simulink model "smMarsRover"  (R2024b)
settings: Solver=VariableStepAuto  StartTime=0.0  StopTime=51  RelTol=1e-3
PreLoadFcn:
  | run_sm
values from neighbouring files (symbols this model uses):
  arm_q0 = [-2.3554 -125.9144   49.8193 -175.7336  177.6446  180.0000]    [sm_mars_rover_params.m]
  goal_loc = [roverPath.x(end) roverPath.y(end)]    [sm_mars_rover_params.m]
  Z = fillmissing(Z, 'linear')    [setup.m]
undefined symbols (not defined in the file or in its folder): cameraData, Chassis_L, Chassis_width, eeConfig, Kd, Kd_arm, Kd_steer, Ki, Ki_arm, Ki_steer, Kp, Kp_arm, Kp_steer, Link1, Link2, Link3, R_disc_Link1, rover_accel, roverPath, t1, TrqLoLimit, TrqUpLimit, Wheel1_G, Wheel2_G, Wheel3_G, Wheel4_G, Wheel5_G, Wheel6_G, Wheel_Radius, X, Y
libraries: sm_lib x216, nesl_utility x51, slpidlib x3, simulink x3, robotcorelib x1, robotalgslib x1, simulink_extras x1
(part 1 of 7)
settings Model: Creator=dipayan  LastModifiedBy=dipayan

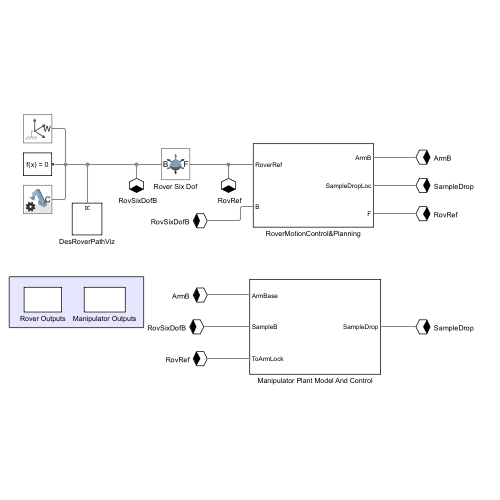
[thumbnail: Simulink's stored preview of the top-level diagram]
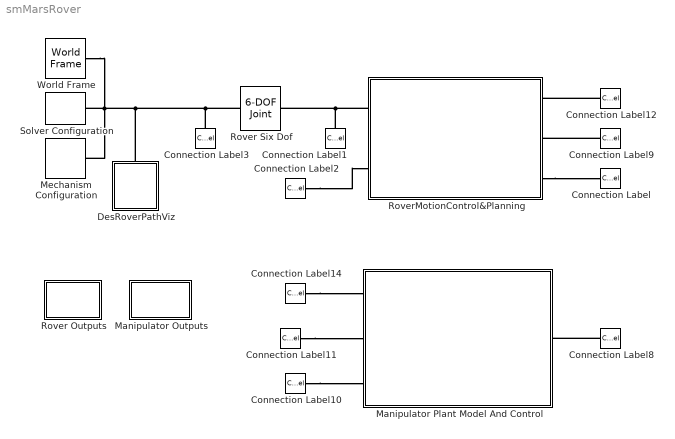
== system smMarsRover ==
  Connection Label : ConnectionLabel  Label=RovRef
  Connection Label1 : ConnectionLabel  Label=RovRef
  Connection Label10 : ConnectionLabel  Label=RovRef
  Connection Label11 : ConnectionLabel  Label=RovSixDofB
  Connection Label12 : ConnectionLabel  Label=ArmB
  Connection Label14 : ConnectionLabel  Label=ArmB
  Connection Label2 : ConnectionLabel  Label=RovSixDofB
  Connection Label3 : ConnectionLabel  Label=RovSixDofB
  Connection Label8 : ConnectionLabel  Label=SampleDrop
  Connection Label9 : ConnectionLabel  Label=SampleDrop
  DesRoverPathViz : Subsystem
  Manipulator Outputs : Subsystem
  Manipulator Plant Model And Control : Subsystem
  Mechanism Configuration : sm_lib/Utilities/Mechanism Configuration  UniformGravity=Constant  GravityVector=[0 0 -3.72076]  GravityVectorUnits=m/s^2  LinearizationDelta=0.001  JointModeTransitionNonlinearIterations=2
  Rover Outputs : Subsystem
  Rover Six Dof : sm_lib/Joints/6-DOF Joint  JointMode=Normal  CompositeWrenchDir=FollowerOnBase  CompositeWrenchFrame=BaseFrame  SenseConstraintForce=off  SenseConstraintTorque=off  SenseTotalForce=off  SenseTotalTorque=off  PxPositionTargetSpecify=on  PxPositionTargetPriority=High  PxPositionTargetValue=roverPath.x(1)  PxPositionTargetValueUnits=m  PxVelocityTargetSpecify=off  PxVelocityTargetPriority=High  PxVelocityTargetValue=0  PxVelocityTargetValueUnits=m/s  PxEquilibriumPosition=0  PxEquilibriumPositionUnits=m  PxSpringStiffness=0  PxSpringStiffnessUnits=N/m  PxDampingCoefficient=0  PxDampingCoefficientUnits=N/(m/s)  PxLowerLimitSpecify=off  PxLowerLimitBound=-1  PxLowerLimitBoundUnits=m  PxLowerLimitStiffness=1e6  PxLowerLimitStiffnessUnits=N/m  PxLowerLimitDamping=1e3  PxLowerLimitDampingUnits=N/(m/s)  PxLowerLimitTransitionRegionWidth=1e-4  PxLowerLimitTransitionRegionWidthUnits=m  PxUpperLimitSpecify=off  PxUpperLimitBound=1  PxUpperLimitBoundUnits=m  PxUpperLimitStiffness=1e6  PxUpperLimitStiffnessUnits=N/m  PxUpperLimitDamping=1e3  PxUpperLimitDampingUnits=N/(m/s)  PxUpperLimitTransitionRegionWidth=1e-4  PxUpperLimitTransitionRegionWidthUnits=m  PxTorqueActuationMode=NoTorque  PxMotionActuationMode=ComputedMotion  PxSensePosition=off  PxSenseVelocity=off  PxSenseAcceleration=off  PxSenseTorqueForce=off  PxSenseLowerLimitTorqueForce=off  PxSenseUpperLimitTorqueForce=off  PyPositionTargetSpecify=on  PyPositionTargetPriority=High  PyPositionTargetValue=roverPath.y(1)  PyPositionTargetValueUnits=m  PyVelocityTargetSpecify=off  PyVelocityTargetPriority=High  PyVelocityTargetValue=-2  PyVelocityTargetValueUnits=m/s  PyEquilibriumPosition=0  PyEquilibriumPositionUnits=m  PySpringStiffness=0  PySpringStiffnessUnits=N/m  PyDampingCoefficient=0  PyDampingCoefficientUnits=N/(m/s)  PyLowerLimitSpecify=off  PyLowerLimitBound=-1  PyLowerLimitBoundUnits=m  PyLowerLimitStiffness=1e6  PyLowerLimitStiffnessUnits=N/m  PyLowerLimitDamping=1e3  PyLowerLimitDampingUnits=N/(m/s)  PyLowerLimitTransitionRegionWidth=1e-4  PyLowerLimitTransitionRegionWidthUnits=m  PyUpperLimitSpecify=off  PyUpperLimitBound=1  PyUpperLimitBoundUnits=m  PyUpperLimitStiffness=1e6  PyUpperLimitStiffnessUnits=N/m  PyUpperLimitDamping=1e3  PyUpperLimitDampingUnits=N/(m/s)  PyUpperLimitTransitionRegionWidth=1e-4  PyUpperLimitTransitionRegionWidthUnits=m  PyTorqueActuationMode=NoTorque  PyMotionActuationMode=ComputedMotion  PySensePosition=off  PySenseVelocity=off  PySenseAcceleration=off  PySenseTorqueForce=off  PySenseLowerLimitTorqueForce=off  PySenseUpperLimitTorqueForce=off  PzPositionTargetSpecify=on  PzPositionTargetPriority=High  PzPositionTargetValue=roverPath.t0.pzOffset  PzPositionTargetValueUnits=m  PzVelocityTargetSpecify=off  PzVelocityTargetPriority=High  PzVelocityTargetValue=0  PzVelocityTargetValueUnits=m/s  PzEquilibriumPosition=0  PzEquilibriumPositionUnits=m  PzSpringStiffness=0  PzSpringStiffnessUnits=N/m  PzDampingCoefficient=0  PzDampingCoefficientUnits=N/(m/s)  PzLowerLimitSpecify=off  PzLowerLimitBound=-1  PzLowerLimitBoundUnits=m  PzLowerLimitStiffness=1e6  PzLowerLimitStiffnessUnits=N/m  PzLowerLimitDamping=1e3  PzLowerLimitDampingUnits=N/(m/s)  PzLowerLimitTransitionRegionWidth=1e-4  PzLowerLimitTransitionRegionWidthUnits=m  PzUpperLimitSpecify=off  PzUpperLimitBound=1  PzUpperLimitBoundUnits=m  PzUpperLimitStiffness=1e6  PzUpperLimitStiffnessUnits=N/m  PzUpperLimitDamping=1e3  PzUpperLimitDampingUnits=N/(m/s)  PzUpperLimitTransitionRegionWidth=1e-4  PzUpperLimitTransitionRegionWidthUnits=m  PzTorqueActuationMode=NoTorque  PzMotionActuationMode=ComputedMotion  PzSensePosition=off  PzSenseVelocity=off  PzSenseAcceleration=off  PzSenseTorqueForce=off  PzSenseLowerLimitTorqueForce=off  PzSenseUpperLimitTorqueForce=off  SphPositionTargetSpecify=on  SphPositionTargetPriority=High  SphPositionTargetRotationMethod=RotationSequence  SphPositionTargetFollAlignAxisA=+X  SphPositionTargetBaseAlignAxisA=+Y  SphPositionTargetFollAlignAxisB=+Y  SphPositionTargetBaseAlignAxisB=+Z  SphPositionTargetRotationStandardAxis=+X  SphPositionTargetRotationAngle=5  SphPositionTargetRotationAngleUnits=deg  SphPositionTargetRotationArbitraryAxis=[0 0 1]  SphPositionTargetRotationSequenceAxes=FollowerAxes  SphPositionTargetRotationSequence=ZYX  SphPositionTargetRotationSequenceAngles=[roverPath.t0.yaw, roverPath.t0.pitch, roverPath.t0.roll]  SphPositionTargetRotationSequenceAnglesUnits=rad  SphPositionTargetRotationMatrix=[1 0 0; 0 1 0; 0 0 1]  SphPositionTargetQuaternion=[1 0 0 0]  SphVelocityTargetSpecify=off  SphVelocityTargetPriority=High  SphVelocityTargetValue=[0 0 45]  SphVelocityTargetValueUnits=deg/s  SphVelocityTargetInFollowerFrame=on  SphEqPosRotationMethod=None  SphEqPosFollAlignAxisA=+X  SphEqPosBaseAlignAxisA=+Y  SphEqPosFollAlignAxisB=+Y  SphEqPosBaseAlignAxisB=+Z  SphEqPosRotationStandardAxis=+Z  SphEqPosRotationAngle=0.0  SphEqPosRotationAngleUnits=deg  SphEqPosRotationArbitraryAxis=[0 0 1]  SphEqPosRotationSequenceAxes=FollowerAxes  SphEqPosRotationSequence=XYX  SphEqPosRotationSequenceAngles=[0 0 0]  SphEqPosRotationSequenceAnglesUnits=deg  SphEqPosRotationMatrix=[1 0 0; 0 1 0; 0 0 1]  SphEqPosQuaternion=[1 0 0 0]  SphSpringStiffness=0  SphSpringStiffnessUnits=m*N/deg  SphDampingCoefficient=0  SphDampingCoefficientUnits=m*s*N/deg  SphLowerLimitSpecify=off  SphLowerLimitBound=15  SphLowerLimitBoundUnits=deg  SphLowerLimitStiffness=1e4  SphLowerLimitStiffnessUnits=N*m/deg  SphLowerLimitDamping=10  SphLowerLimitDampingUnits=N*m/(deg/s)  SphLowerLimitTransitionRegionWidth=0.1  SphLowerLimitTransitionRegionWidthUnits=deg  SphUpperLimitSpecify=off  SphUpperLimitBound=45  SphUpperLimitBoundUnits=deg  SphUpperLimitStiffness=1e4  SphUpperLimitStiffnessUnits=N*m/deg  SphUpperLimitDamping=10  SphUpperLimitDampingUnits=N*m/(deg/s)  SphUpperLimitTransitionRegionWidth=0.1  SphUpperLimitTransitionRegionWidthUnits=deg  SphTorqueActuationMode=NoTorque  SphActuateTorqueX=off  SphActuateTorqueY=off  SphActuateTorqueZ=off  SphActuateTorque=off  SphActuationFrame=BaseFrame  SphSensePosition=off  SphSenseVelocityX=off  SphSenseVelocityY=off  SphSenseVelocityZ=off  SphSenseVelocity=off  SphSenseAccelerationX=off  SphSenseAccelerationY=off  SphSenseAccelerationZ=off  SphSenseAcceleration=off  SphSenseLowerLimitTorqueMag=off  SphSenseUpperLimitTorqueMag=off  SphSensingFrame=FollowerFrame
  RoverMotionControl&Planning : Subsystem
  Solver Configuration : nesl_utility/Solver Configuration  PhysicalDomain=network_engine_domain  SubClassName=solver  LeftPortType=input  RightPortType=generic  Tones=[]  Harmonics=[]  SimulateNoise=off  Profile=off  UseLocalSampling=off  EnableSwitchedLinearOptims=on  FrequencyDomain=off  UseCCode=off  RelTol=0.001  AbsTol=1e-06  MinStep=1e-09  ToWorkspace=off  RevertToSquareIcSolve=off  NumHomotopyIterations=100  PhasorMode=off  PhasorModeNumHarmonics=1  ConsistencySolver=NEWTON_FTOL  IndexReductionMethod=DerivativeReplacement  DoDC=off  ResidualTolerance=1e-09  ConsistencyTolSource=GLOBAL  ConsistencyAbsTol=0.001  ConsistencyRelTol=0.001  ConsistencyTolFactor=0.001  UseLocalSolver=off  LocalSolverChoice=NE_BACKWARD_EULER_ADVANCER  ResolveIndetEquations=on  FunctionEvalNumThread=1  LocalSolverSampleTime=0.001  DoFixedCost=off  MaxNonlinIter=3  MaxModeIter=2  ComputeImpulses=off  ImpulseIterations=2  LinearAlgebra=auto  LinearAlgebraNumThread=0  EquationFormulation=NE_TIME_EF  DelaysMemoryBudget=1024  AutomaticFiltering=on  FilteringTimeConstant=0.001  PartitionStorageMethod=AS_NEEDED  PartitionMemoryBudget=1024  PartitionMethod=FAST  MultibodyUseLocalSolver=off  MultibodyLocalSolverChoice=ODE1  MultibodyLocalSolverSampleTime=0.001
  World Frame : sm_lib/Frames and Transforms/World Frame
  connections:
  Solver Configuration/RConn1 -- Connection Label3/LConn1 -- Rover Six Dof/LConn1 -- DesRoverPathViz/LConn1 -- World Frame/RConn1 -- Mechanism Configuration/RConn1
  RoverMotionControl&Planning/LConn1 -- Connection Label1/LConn1 -- Rover Six Dof/RConn1
  RoverMotionControl&Planning/RConn3 -- Connection Label/LConn1
  Connection Label12/LConn1 -- RoverMotionControl&Planning/RConn1
  Connection Label9/LConn1 -- RoverMotionControl&Planning/RConn2
  Connection Label2/LConn1 -- RoverMotionControl&Planning/LConn2
  Connection Label14/LConn1 -- Manipulator Plant Model And Control/LConn1
  Connection Label11/LConn1 -- Manipulator Plant Model And Control/LConn2
  Connection Label10/LConn1 -- Manipulator Plant Model And Control/LConn3
  Connection Label8/LConn1 -- Manipulator Plant Model And Control/RConn1

== system smMarsRover/DesRoverPathViz ==
  Desired Path Viz : sm_lib/Curves and Surfaces/Point Cloud  CoordinatesMatrix=pointCloud  CoordinatesMatrixUnits=m  GraphicType=MarkerCloud  GraphicSphereRadius=0.05  GraphicSphereRadiusUnits=m  GraphicVisPropType=SimpleVisualProperties  GraphicDiffuseColor=[0 0 1]  GraphicOpacity=0.5  GraphicSpecularColor=[0.5 0.5 0.5 1.0]  GraphicAmbientColor=[0.15 0.15 0.15 1.0]  GraphicEmissiveColor=[0.0 0.0 0.0 1.0]  GraphicShininess=75
  Rigid Transform6 : sm_lib/Frames and Transforms/Rigid Transform  RotationMethod=None  FollAlignAxisA=+X  BaseAlignAxisA=+Y  FollAlignAxisB=+Y  BaseAlignAxisB=+Z  RotationStandardAxis=+X  RotationAngle=90  RotationAngleUnits=deg  RotationArbitraryAxis=[0 0 1]  RotationSequenceAxes=FollowerAxes  RotationSequence=XYX  RotationSequenceAngles=[0 0 0]  RotationSequenceAnglesUnits=deg  RotationMatrix=[1 0 0; 0 1 0; 0 0 1]  Quaternion=[1 0 0 0]  TranslationMethod=Cartesian  TranslationCartesianOffset=[0 0 roverPath.Offset_vis_z]  TranslationCartesianOffsetUnits=m  TranslationStandardAxis=+Z  TranslationStandardOffset=1.85  TranslationStandardOffsetUnits=m  TranslationROffset=0  TranslationROffsetUnits=m  TranslationThetaOffset=0  TranslationThetaOffsetUnits=deg  TranslationZOffset=0  TranslationZOffsetUnits=m
  Spline : sm_lib/Curves and Surfaces/Spline  DataPoints=pointCloud  DataPointsUnits=m  EndConditionType=Natural  GraphicType=FromGeometry  MarkerShape=Sphere  MarkerSize=10  GraphicVisPropType=SimpleVisualProperties  GraphicDiffuseColor=[0 0.4471 0.7412]  GraphicOpacity=0.5  GraphicSpecularColor=[0.5 0.5 0.5 1.0]  GraphicAmbientColor=[0.15 0.15 0.15 1.0]  GraphicEmissiveColor=[0.0 0.0 0.0 1.0]  GraphicShininess=75
  R : PMIOPort  Side=Left
  connections:
  Desired Path Viz/LConn1 -- Rigid Transform6/RConn1 -- Spline/LConn1
  R/RConn1 -- Rigid Transform6/LConn1

== system smMarsRover/Manipulator Outputs ==
  ManipulatorJointActuatorTrqs : Scope  NumInputPorts=6
  ManipulatorJointAngles : Scope  NumInputPorts=6
  SelectSignal4 : Subsystem
  SelectSignal5 : Subsystem
  wires:
  SelectSignal4/5(Out4) -> ManipulatorJointAngles/5
  SelectSignal5/3(Out3) -> ManipulatorJointActuatorTrqs/3
  SelectSignal4/2(Out2) -> ManipulatorJointAngles/2
  SelectSignal4/1(Out1) -> ManipulatorJointAngles/1
  SelectSignal5/2(Out2) -> ManipulatorJointActuatorTrqs/2
  SelectSignal4/6(Out6) -> ManipulatorJointAngles/6
  SelectSignal5/4(Out5) -> ManipulatorJointActuatorTrqs/4
  SelectSignal4/3(Out3) -> ManipulatorJointAngles/3
  SelectSignal5/1(Out1) -> ManipulatorJointActuatorTrqs/1
  SelectSignal5/5(Out4) -> ManipulatorJointActuatorTrqs/5
  SelectSignal4/4(Out5) -> ManipulatorJointAngles/4
  [DesiredJointAngles] -> SelectSignal4/1(In1)
  [JointActuatorTrqs] -> SelectSignal5/1(In1)
  [ActJointAngles] -> SelectSignal4/2(In2)
  SelectSignal5/6(Out6) -> ManipulatorJointActuatorTrqs/6

== system smMarsRover/Manipulator Plant Model And Control ==
  " Trajectory Planner" : Subsystem
  Add : Sum  Inputs=+-
  ArmLock : Subsystem
  End Effector Sense : Subsystem
  PID Control : slpidlib/PID Controller  Controller=PID  Form=Parallel  TimeDomain=Continuous-time  UseExternalTs=off  SampleTime=-1  IntegratorMethod=Forward Euler  FilterMethod=Forward Euler  ControllerParametersSource=internal  P=Kp_arm  I=Ki_arm  UseKiTs=off  D=Kd_arm  UseExternalDerivativeSource=off  N=100  UseFilter=on  TunerSelectOption=Transfer Function Based (PID Tuner App)  InitialConditionSource=internal  InitialConditionForIntegrator=0  InitialConditionForFilter=0  DifferentiatorICPrevScaledInput=0  ExternalReset=none  TrackingMode=off  Kt=1  LimitOutput=off  SatLimitsSource=internal  UpperSaturationLimit=inf  LowerSaturationLimit=-inf  LinearizeAsGain=on  AntiWindupMode=none  Kb=1  LimitIntegrator=off  UpperIntegratorSaturationLimit=inf  LowerIntegratorSaturationLimit=-inf  POutMin=[]  POutMax=[]  IOutMin=[]  IOutMax=[]  DOutMin=[]  DOutMax=[]  NOutMin=[]  NOutMax=[]  SumOutMin=[]  SumOutMax=[]  SaturationOutMin=[]  SaturationOutMax=[]  PParamMin=[]  PParamMax=[]  IParamMin=[]  IParamMax=[]  DParamMin=[]  DParamMax=[]  NParamMin=[]  NParamMax=[]  KbParamMin=[]  KbParamMax=[]  KtParamMin=[]  KtParamMax=[]  KbOutMin=[]  KbOutMax=[]  KtOutMin=[]  KtOutMax=[]  IntegratorOutMin=[]  IntegratorOutMax=[]  FilterOutMin=[]  FilterOutMax=[]  SumI1OutMin=[]  SumI1OutMax=[]  SumI2OutMin=[]  SumI2OutMax=[]  SumI3OutMin=[]  SumI3OutMax=[]  SumI4OutMin=[]  SumI4OutMax=[]  SumDOutMin=[]  SumDOutMax=[]  DifferentiatorOutMin=[]  DifferentiatorOutMax=[]  FilterDiffOutCoefMin=[]  FilterDiffOutCoefMax=[]  ReciprocalOutMin=[]  ReciprocalOutMax=[]  SumDenOutMin=[]  SumDenOutMax=[]  SumNumOutMin=[]  SumNumOutMax=[]  DivideOutMin=[]  DivideOutMax=[]  UdiffTsProdOutMin=[]  UdiffTsProdOutMax=[]  NTsProdOutMin=[]  NTsProdOutMax=[]  UintegralTsProdOutMin=[]  UintegralTsProdOutMax=[]  UngainTsProdOutMin=[]  UngainTsProdOutMax=[]  ClampingZeroOutDataTypeStr=Inherit: Inherit via back propagation  ClampingZeroOutMin=[]  ClampingZeroOutMax=[]  FilterDenConstantOutDataTypeStr=Inherit: Inherit via back propagation  FilterDenConstantOutMin=[]  FilterDenConstantOutMax=[]  PCopyOutDataTypeStr=Inherit: Inherit via back propagation  PCopyOutMin=[]  PCopyOutMax=[]  NCopyOutDataTypeStr=Inherit: Inherit via back propagation  NCopyOutMin=[]  NCopyOutMax=[]  IntegratorContinuousStateAttributes=''  IntegratorStateMustResolveToSignalObject=off  IntegratorRTWStateStorageClass=Auto  FilterContinuousStateAttributes=''  FilterStateMustResolveToSignalObject=off  FilterRTWStateStorageClass=Auto  ParallelPVariant=InternalParameters  IdealPVariant=Disabled  IVariant=InternalParameters  DVariant=InternalParameters  IntegratorVariant=Continuous  SatVariant=Disabled  AWVariant=Passthrough  PCopyVariant=Disabled  TRVariant=Disabled  FdbkBlocksVariant=Forward  IdealPFdbkVariant=Disabled  SatFdbkVariant=Disabled  DerivativeFilterVariant=ContFilter  NVariant=InternalParameters  NCopyVariant=Disabled  FilterICVariant=InternalICsFilter  IntegratorICVariant=InternalICs  ExternalResetVariant=Disabled  TRSumVariant=Passthrough  SumFdbkVariant=Disabled  SumVariant=Sum_PID  TsampFilterVariant=InternalTs  TsampNgainVariant=Passthrough  TsampIntegralVariant=Disabled_SignalSpec  ExternalSaturationOutDataTypeStr=Inherit: Same as second input  DerivativeSourceVariant=ErrorSignal  PreIntVariant=InternalPreInt
  Rover Arm : Subsystem
      settings: PortSchema="{\"entries\":[{\"content\":{\"sides\":[{\"content\":{\"connectorIds\":[\"In1\"]},\"type\":\"ConnectorPlacement.EquallySpacedRectSide\",\"uuid\":\"44c8adb7-00ac-400a-98ed-ead5e12ad105\"},{\"content\":{\"connectorIds\":[\"Out1\"],\"side\":\"RIGHT\"},\"type\":\"ConnectorPlacement.EquallySpacedRectSide\",\"uuid\":\"fdc7bd8f-ace2-488d-8919-cf5c650dd1d7\"},{\"content\":{\"connectorIds\":[\"LConn1\",\"LConn2\"],\"side\":\"TOP\"},\"type\":\"ConnectorPlacement.EquallySpacedRectSide\",\"uuid\":\"e6b89b0c-12bb-4698-b60e-60c64a8f3314\"}]},\"type\":\"ConnectorPlacement.EquallySpacedConnector\",\"uuid\":\"42e45278-5e8a-4850-9160-494ec176052c\"}],\"packageUris\":[\"http://schema.mathworks.com/mf0/Connector/R2020b\"],\"version\":\"1.0\"}"
      mask Display: image('rover_manip_subsys_1.JPG');
  Sample Interaction Logic : Subsystem
      mask Display: image('sample_1.JPG');
  Sample Loc Sense : Subsystem
  ArmBase : PMIOPort  Side=Left
  SampleB : PMIOPort  Port=2  Side=Left
  ToArmLock : PMIOPort  Port=3  Side=Left
  SampleDrop : PMIOPort  Port=4  Side=Right
  tag scope: ActJointAngles=global, DesiredJointAngles=global, JointActuatorTrqs=global
  wires:
  Add/1 -> PID Control/1
  Rover Arm/1(JointAngles) -> " Trajectory Planner"/2(ActJointAngles), Add/2, [ActJointAngles]
  " Trajectory Planner"/1(DesiredJointAngles) -> [DesiredJointAngles], Add/1
  PID Control/1 -> [JointActuatorTrqs], Rover Arm/1(ActuatorTrqs)
  Sample Loc Sense/1(SamplePos) -> " Trajectory Planner"/1(SampleLocation)
  connections:
  Rover Arm/LConn2 -- Sample Interaction Logic/LConn2 -- ArmLock/RConn1 -- End Effector Sense/RConn1
  Rover Arm/LConn1 -- ArmBase/RConn1 -- Sample Loc Sense/LConn1 -- End Effector Sense/LConn1
  SampleB/RConn1 -- Sample Interaction Logic/LConn3
  Sample Loc Sense/RConn1 -- Sample Interaction Logic/LConn1
  SampleDrop/RConn1 -- Sample Interaction Logic/RConn1
  ToArmLock/RConn1 -- ArmLock/LConn1

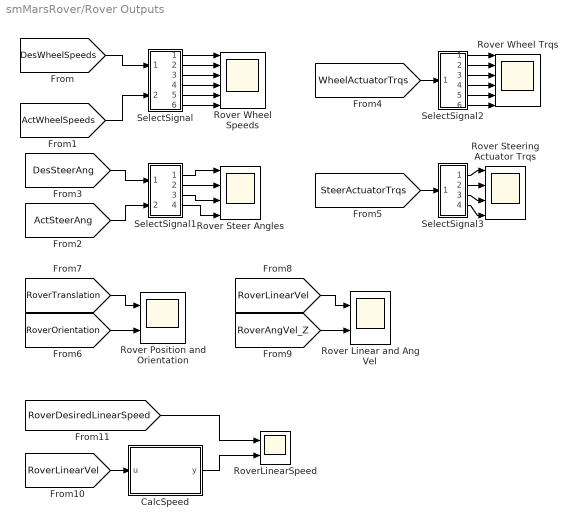
== system smMarsRover/Rover Outputs ==
  CalcSpeed : MATLAB Function  TreatAsAtomicUnit=on
  Rover Linear and Ang Vel : Scope  NumInputPorts=2
  Rover Position and Orientation : Scope  NumInputPorts=2
  Rover Steer Angles : Scope  NumInputPorts=4
  Rover Steering Actuator Trqs : Scope  NumInputPorts=4
  Rover Wheel Speeds : Scope  NumInputPorts=6
  Rover Wheel Trqs : Scope  NumInputPorts=6
  RoverLinearSpeed : Scope  NumInputPorts=2
  SelectSignal : Subsystem
  SelectSignal1 : Subsystem
  SelectSignal2 : Subsystem
  SelectSignal3 : Subsystem
  wires:
  CalcSpeed/1(y) -> RoverLinearSpeed/2
  SelectSignal3/1(Out1) -> Rover Steering Actuator Trqs/1
  [RoverLinearVel] -> CalcSpeed/1(u)
  [RoverAngVel_Z] -> Rover Linear and Ang Vel/2
  [RoverLinearVel] -> Rover Linear and Ang Vel/1
  [DesWheelSpeeds] -> SelectSignal/1(In1)
  SelectSignal2/4(Out4) -> Rover Wheel Trqs/4
  [WheelActuatorTrqs] -> SelectSignal2/1(In1)
  SelectSignal1/2(Out2) -> Rover Steer Angles/2
  [RoverTranslation] -> Rover Position and Orientation/1
  SelectSignal3/2(Out2) -> Rover Steering Actuator Trqs/2
  SelectSignal3/3(Out3) -> Rover Steering Actuator Trqs/3
  [DesSteerAng] -> SelectSignal1/1(In1)
  SelectSignal2/3(Out3) -> Rover Wheel Trqs/3
  [RoverOrientation] -> Rover Position and Orientation/2
  SelectSignal3/4(Out5) -> Rover Steering Actuator Trqs/4
  SelectSignal2/6(Out6) -> Rover Wheel Trqs/6
  SelectSignal/3(Out3) -> Rover Wheel Speeds/3
  SelectSignal2/5(Out5) -> Rover Wheel Trqs/5
  SelectSignal/1(Out1) -> Rover Wheel Speeds/1
  SelectSignal/6(Out6) -> Rover Wheel Speeds/6
  [ActWheelSpeeds] -> SelectSignal/2(In2)
  SelectSignal2/1(Out1) -> Rover Wheel Trqs/1
  SelectSignal1/4(Out5) -> Rover Steer Angles/4
  [ActSteerAng] -> SelectSignal1/2(In2)
  SelectSignal/2(Out2) -> Rover Wheel Speeds/2
  [SteerActuatorTrqs] -> SelectSignal3/1(In1)
  SelectSignal/5(Out4) -> Rover Wheel Speeds/5
  SelectSignal2/2(Out2) -> Rover Wheel Trqs/2
  SelectSignal/4(Out5) -> Rover Wheel Speeds/4
  SelectSignal1/1(Out1) -> Rover Steer Angles/1
  SelectSignal1/3(Out3) -> Rover Steer Angles/3
  [RoverDesiredLinearSpeed] -> RoverLinearSpeed/1

== system smMarsRover/RoverMotionControl&Planning ==
  Rigid Terrain Surface : Subsystem
      mask Display: image('$imagefile'); % Use "Edit Image" on toolstrip to change.
  "Rover " : Subsystem
      settings: PortSchema="{\"entries\":[{\"content\":{\"sides\":[{\"content\":{\"connectorIds\":[\"LConn1\",\"In1\",\"In2\"]},\"type\":\"ConnectorPlacement.EquallySpacedRectSide\",\"uuid\":\"1e8a3e2b-b3ca-4467-863a-9c237d71771f\"},{\"content\":{\"connectorIds\":[\"RConn1\",\"RConn2\",\"RConn3\",\"Out1\",\"Out2\"],\"side\":\"RIGHT\"},\"type\":\"ConnectorPlacement.EquallySpacedRectSide\",\"uuid\":\"1c304fdb-ff64-4dc8-bd28-208b239a200a\"},{\"content\":{\"connectorIds\":[],\"side\":\"TOP\"},\"type\":\"ConnectorPlacement.EquallySpacedRectSide\",\"uuid\":\"6fd19973-5814-4525-bce6-20dd9c942e44\"}]},\"type\":\"ConnectorPlacement.EquallySpacedConnector\",\"uuid\":\"720db96a-3f3b-4ddd-a986-ea75ab459e47\"}],\"packageUris\":[\"http://schema.mathworks.com/mf0/Connector/R2020b\"],\"version\":\"1.0\"}"
      mask Display: image('$imagefile'); % Use "Edit Image" on toolstrip to change.
  Rover Path Planning And Control : Subsystem
  Rover Pose Sensing : Subsystem
  Steering Controller : Subsystem
  Wheel Speed Controller : Subsystem
  World Frame1 : sm_lib/Frames and Transforms/World Frame
  RoverRef : PMIOPort  Side=Left
  B : PMIOPort  Port=2  Side=Left
  ArmB : PMIOPort  Port=3  Side=Right
  SampleDropLoc : PMIOPort  Port=4  Side=Right
  F : PMIOPort  Port=5  Side=Right
  wires:
  "Rover "/1(ActSteerAng) -> Steering Controller/2(ActSteerAng)
  Rover Pose Sensing/1(Pose) -> Rover Path Planning And Control/1(CurrentPose)
  Rover Path Planning And Control/2(DesWheelSpeeds) -> Wheel Speed Controller/1(DesWheelSpeeds)
  "Rover "/2(ActWheelSpeeds) -> Wheel Speed Controller/2(ActWheelSpeed)
  Rover Pose Sensing/2(vSpeed) -> Rover Path Planning And Control/2(vSpeed)
  Steering Controller/1(SteerTrqs) -> "Rover "/1(SteeringTrqs)
  Rover Path Planning And Control/1(DesSteerAngs) -> Steering Controller/1(DesSteerAng)
  Wheel Speed Controller/1(WheelTrqs) -> "Rover "/2(WheelTrqs)
  connections:
  Rigid Terrain Surface/LConn1 -- "Rover "/RConn3
  SampleDropLoc/RConn1 -- "Rover "/RConn2
  B/RConn1 -- Rover Pose Sensing/LConn1
  World Frame1/RConn1 -- Rigid Terrain Surface/RConn1
  ArmB/RConn1 -- "Rover "/RConn1
  F/RConn1 -- Rover Pose Sensing/RConn1
  RoverRef/RConn1 -- "Rover "/LConn1

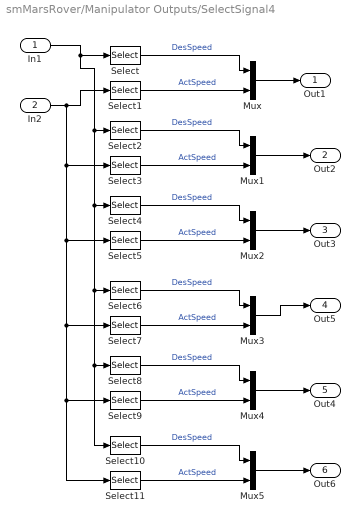
== system smMarsRover/Manipulator Outputs/SelectSignal4 ==
  In1 : Inport
  In2 : Inport  Port=2
  Mux{,1..5} (6 alike) : Mux  Inputs=2
  Select : Selector  InputPortWidth=6  IndexOptions=Index vector (dialog)  Indices=1  OutputSizes=1
  Select1 : Selector  InputPortWidth=6  IndexOptions=Index vector (dialog)  Indices=1  OutputSizes=1
  Select10 : Selector  InputPortWidth=6  IndexOptions=Index vector (dialog)  Indices=6  OutputSizes=1
  Select11 : Selector  InputPortWidth=6  IndexOptions=Index vector (dialog)  Indices=6  OutputSizes=1
  Select2 : Selector  InputPortWidth=6  IndexOptions=Index vector (dialog)  Indices=2  OutputSizes=1
  Select3 : Selector  InputPortWidth=6  IndexOptions=Index vector (dialog)  Indices=2  OutputSizes=1
  Select4 : Selector  InputPortWidth=6  IndexOptions=Index vector (dialog)  Indices=3  OutputSizes=1
  Select5 : Selector  InputPortWidth=6  IndexOptions=Index vector (dialog)  Indices=3  OutputSizes=1
  Select6 : Selector  InputPortWidth=6  IndexOptions=Index vector (dialog)  Indices=4  OutputSizes=1
  Select7 : Selector  InputPortWidth=6  IndexOptions=Index vector (dialog)  Indices=4  OutputSizes=1
  Select8 : Selector  InputPortWidth=6  IndexOptions=Index vector (dialog)  Indices=5  OutputSizes=1
  Select9 : Selector  InputPortWidth=6  IndexOptions=Index vector (dialog)  Indices=5  OutputSizes=1
  Out1 : Outport
  Out2 : Outport  Port=2
  Out3 : Outport  Port=3
  Out5 : Outport  Port=4
  Out4 : Outport  Port=5
  Out6 : Outport  Port=6
  wires:
  Select11/1 -> Mux5/2  "ActSpeed"
  Mux5/1 -> Out6/1
  Select10/1 -> Mux5/1  "DesSpeed"
  Select8/1 -> Mux4/1  "DesSpeed"
  Mux4/1 -> Out4/1
  Select9/1 -> Mux4/2  "ActSpeed"
  Select7/1 -> Mux3/2  "ActSpeed"
  Mux3/1 -> Out5/1
  Select6/1 -> Mux3/1  "DesSpeed"
  Select4/1 -> Mux2/1  "DesSpeed"
  Mux2/1 -> Out3/1
  Select5/1 -> Mux2/2  "ActSpeed"
  Select3/1 -> Mux1/2  "ActSpeed"
  Mux1/1 -> Out2/1
  Select2/1 -> Mux1/1  "DesSpeed"
  In2/1 -> Select1/1, Select3/1, Select5/1, Select7/1, Select9/1, Select11/1
  Select/1 -> Mux/1  "DesSpeed"
  In1/1 -> Select/1, Select2/1, Select4/1, Select6/1, Select8/1, Select10/1
  Mux/1 -> Out1/1
  Select1/1 -> Mux/2  "ActSpeed"

== system smMarsRover/Manipulator Outputs/SelectSignal5 ==
  In1 : Inport
  Select : Selector  InputPortWidth=6  IndexOptions=Index vector (dialog)  Indices=1  OutputSizes=1
  Select10 : Selector  InputPortWidth=6  IndexOptions=Index vector (dialog)  Indices=6  OutputSizes=1
  Select2 : Selector  InputPortWidth=6  IndexOptions=Index vector (dialog)  Indices=2  OutputSizes=1
  Select4 : Selector  InputPortWidth=6  IndexOptions=Index vector (dialog)  Indices=3  OutputSizes=1
  Select6 : Selector  InputPortWidth=6  IndexOptions=Index vector (dialog)  Indices=4  OutputSizes=1
  Select8 : Selector  InputPortWidth=6  IndexOptions=Index vector (dialog)  Indices=5  OutputSizes=1
  Transfer Fcn{1..6} (6 alike) : TransferFcn  Denominator=[0.1 1]
  Out1 : Outport
  Out2 : Outport  Port=2
  Out3 : Outport  Port=3
  Out5 : Outport  Port=4
  Out4 : Outport  Port=5
  Out6 : Outport  Port=6
  wires:
  Select10/1 -> Transfer Fcn5/1
  Select8/1 -> Transfer Fcn1/1
  Select6/1 -> Transfer Fcn2/1
  Select4/1 -> Transfer Fcn3/1
  Select2/1 -> Transfer Fcn4/1
  Select/1 -> Transfer Fcn6/1
  In1/1 -> Select10/1, Select8/1, Select6/1, Select4/1, Select2/1, Select/1
  Transfer Fcn6/1 -> Out1/1
  Transfer Fcn4/1 -> Out2/1
  Transfer Fcn3/1 -> Out3/1
  Transfer Fcn2/1 -> Out5/1
  Transfer Fcn1/1 -> Out4/1
  Transfer Fcn5/1 -> Out6/1

== system smMarsRover/Manipulator Plant Model And Control/ Trajectory Planner ==
  SampleLocation : Inport
  ActJointAngles : Inport  Port=2
  Constant : Constant  Value="[-2.2294 -125.2918   50.0575 -175.3493  177.7706  180.0000]"
  Delay : Delay
  Planner Subsystem : Subsystem
  SampleDropOffCmdLogic : Subsystem
  SampleLoc wrt arm base : Subsystem
  SamplePickUpCmdLogic : Subsystem
  Stop Simulation : Stop
  Switch : Switch  Criteria=u2 > Threshold  SaturateOnIntegerOverflow=off  InputSameDT=off
  DesiredJointAngles : Outport
  tag scope: ArmEnable=global, SampleDropOffFlag=global, SamplePickFlag=global
  wires:
  [RoverAtGoal] -> Planner Subsystem/Enable, Delay/1, SampleLoc wrt arm base/1(Enable)
  Switch/1 -> DesiredJointAngles/1
  Constant/1 -> Switch/3
  SampleDropOffCmdLogic/1(Out1) -> [SampleDropOffFlag]
  SamplePickUpCmdLogic/1(Out1) -> [SamplePickFlag]
  Delay/1 -> [ArmEnable], Switch/2
  ActJointAngles/1 -> Planner Subsystem/1(ActJointAngles)
  SampleLoc wrt arm base/1(SamplePos) -> Planner Subsystem/2(SamplePosition)
  Planner Subsystem/2(SamplePickCmd) -> SamplePickUpCmdLogic/1(u)
  Planner Subsystem/3(SampleDropCmd) -> SampleDropOffCmdLogic/1(u)
  [samplePickedSense] -> Planner Subsystem/3(IsSamplePicked)
  [sampleStoredSense] -> Planner Subsystem/4(IsSampleCollected)
  Planner Subsystem/1(DesJointAngles) -> Switch/1
  SampleLocation/1 -> SampleLoc wrt arm base/2(SampleLoc)
  Planner Subsystem/4(stop) -> Stop Simulation/1

== system smMarsRover/Manipulator Plant Model And Control/ArmLock ==
  note: Open arm lock by disengaging the Pristmatic joint when ArmEnable signal is true
  Constant1 : Constant  Value=-1
  Constant2 : Constant  Value=0
  Delay : Delay
  Rigid Transform : sm_lib/Frames and Transforms/Rigid Transform  RotationMethod=None  FollAlignAxisA=+X  BaseAlignAxisA=+Y  FollAlignAxisB=+Y  BaseAlignAxisB=+Z  RotationStandardAxis=+Z  RotationAngle=0.0  RotationAngleUnits=deg  RotationArbitraryAxis=[0 0 1]  RotationSequenceAxes=FollowerAxes  RotationSequence=XYX  RotationSequenceAngles=[0 0 0]  RotationSequenceAnglesUnits=deg  RotationMatrix=[1 0 0; 0 1 0; 0 0 1]  Quaternion=[1 0 0 0]  TranslationMethod=StandardAxis  TranslationCartesianOffset=[0 0 0]  TranslationCartesianOffsetUnits=m  TranslationStandardAxis=+Z  TranslationStandardOffset=-0.38  TranslationStandardOffsetUnits=m  TranslationROffset=0  TranslationROffsetUnits=m  TranslationThetaOffset=0  TranslationThetaOffsetUnits=deg  TranslationZOffset=0  TranslationZOffsetUnits=m
  Rigid Transform1 : sm_lib/Frames and Transforms/Rigid Transform  RotationMethod=StandardAxis  FollAlignAxisA=+X  BaseAlignAxisA=+Y  FollAlignAxisB=+Y  BaseAlignAxisB=+Z  RotationStandardAxis=+Z  RotationAngle=90  RotationAngleUnits=deg  RotationArbitraryAxis=[0 0 1]  RotationSequenceAxes=FollowerAxes  RotationSequence=XYX  RotationSequenceAngles=[0 0 0]  RotationSequenceAnglesUnits=deg  RotationMatrix=[1 0 0; 0 1 0; 0 0 1]  Quaternion=[1 0 0 0]  TranslationMethod=Cartesian  TranslationCartesianOffset=[0.6000 0.4853 0.3652]  TranslationCartesianOffsetUnits=m  TranslationStandardAxis=+Z  TranslationStandardOffset=0  TranslationStandardOffsetUnits=m  TranslationROffset=0  TranslationROffsetUnits=m  TranslationThetaOffset=0  TranslationThetaOffsetUnits=deg  TranslationZOffset=0  TranslationZOffsetUnits=m
  SPrismatic Joint : sm_lib/Joints/Prismatic Joint  JointMode=ProvidedByInput  CompositeWrenchDir=FollowerOnBase  CompositeWrenchFrame=BaseFrame  SenseConstraintForce=off  SenseConstraintTorque=off  SenseTotalForce=off  SenseTotalTorque=off  PositionTargetSpecify=off  PositionTargetPriority=High  PositionTargetValue=0  PositionTargetValueUnits=m  VelocityTargetSpecify=off  VelocityTargetPriority=High  VelocityTargetValue=0  VelocityTargetValueUnits=m/s  EquilibriumPosition=0  EquilibriumPositionUnits=m  SpringStiffness=0  SpringStiffnessUnits=N/m  DampingCoefficient=0  DampingCoefficientUnits=N/(m/s)  LowerLimitSpecify=on  LowerLimitBound=0  LowerLimitBoundUnits=m  LowerLimitStiffness=1e6  LowerLimitStiffnessUnits=N/m  LowerLimitDamping=1e3  LowerLimitDampingUnits=N/(m/s)  LowerLimitTransitionRegionWidth=1e-4  LowerLimitTransitionRegionWidthUnits=m  UpperLimitSpecify=off  UpperLimitBound=1  UpperLimitBoundUnits=m  UpperLimitStiffness=1e6  UpperLimitStiffnessUnits=N/m  UpperLimitDamping=1e3  UpperLimitDampingUnits=N/(m/s)  UpperLimitTransitionRegionWidth=1e-4  UpperLimitTransitionRegionWidthUnits=m  TorqueActuationMode=NoTorque  MotionActuationMode=ComputedMotion  SensePosition=off  SenseVelocity=off  SenseAcceleration=off  SenseTorqueForce=off  SenseLowerLimitTorqueForce=off  SenseUpperLimitTorqueForce=off
  Simulink-PS Converter : nesl_utility/Simulink-PS Converter  PhysicalDomain=network_engine_domain  SubClassName=ps_input  LeftPortType=input  RightPortType=output  PseudoPeriodic=off  Frequencies=[]  NoiseDistribution=none  NoiseParameters=[]  Unit=1  AffineConversion=off  FilteringAndDerivatives=provide  SimscapeFilterOrder=1  InputFilterTimeConstant=0.001  UdotUserProvided=0
  Switch1 : Switch  Criteria=u2 > Threshold  SaturateOnIntegerOverflow=off  InputSameDT=off
  Conn1 : PMIOPort  Side=Right
  Conn2 : PMIOPort  Port=2  Side=Left
  wires:
  Constant1/1 -> Switch1/1
  Switch1/1 -> Simulink-PS Converter/1
  Constant2/1 -> Switch1/3
  [ArmEnable] -> Delay/1
  Delay/1 -> Switch1/2
  connections:
  Rigid Transform1/LConn1 -- Rigid Transform/RConn1
  SPrismatic Joint/LConn1 -- Rigid Transform1/RConn1
  Simulink-PS Converter/RConn1 -- SPrismatic Joint/LConn2
  Conn1/RConn1 -- SPrismatic Joint/RConn1
  Rigid Transform/LConn1 -- Conn2/RConn1

== system smMarsRover/Manipulator Plant Model And Control/End Effector Sense ==
  Mux1 : Mux  Inputs=3
  PS-Simulink Converter6 : nesl_utility/PS-Simulink Converter  PhysicalDomain=network_engine_domain  SubClassName=ps_output  LeftPortType=input  RightPortType=output  PseudoPeriodic=off  Frequencies=[]  VectorFormat=1-D array  Unit=inherit  AffineConversion=off
  PS-Simulink Converter7 : nesl_utility/PS-Simulink Converter  PhysicalDomain=network_engine_domain  SubClassName=ps_output  LeftPortType=input  RightPortType=output  PseudoPeriodic=off  Frequencies=[]  VectorFormat=1-D array  Unit=inherit  AffineConversion=off
  PS-Simulink Converter8 : nesl_utility/PS-Simulink Converter  PhysicalDomain=network_engine_domain  SubClassName=ps_output  LeftPortType=input  RightPortType=output  PseudoPeriodic=off  Frequencies=[]  VectorFormat=1-D array  Unit=inherit  AffineConversion=off
  Terminator : Terminator
  Transform Sensor : sm_lib/Frames and Transforms/Transform Sensor  MeasurementFrame=Base  RotationSequence=XYX  SenseAngle=off  SenseAxis=off  SenseQ=off  SenseR=off  SenseRotationSequence=off  SenseOmegaX=off  SenseOmegaY=off  SenseOmegaZ=off  SenseOmega=off  SenseQDot=off  SenseRDot=off  SenseRotationSequenceDot=off  SenseAlphaX=off  SenseAlphaY=off  SenseAlphaZ=off  SenseAlpha=off  SenseQDDot=off  SenseRDDot=off  SenseX=on  SenseY=on  SenseZ=on  SenseXYZ=off  SenseRad=off  SenseAzim=off  SenseDist=off  SenseInc=off  SenseXDot=off  SenseYDot=off  SenseZDot=off  SenseXYZDot=off  SenseRadDot=off  SenseAzimDot=off  SenseDistDot=off  SenseIncDot=off  SenseXDDot=off  SenseYDDot=off  SenseZDDot=off  SenseXYZDDot=off  SenseRadDDot=off  SenseAzimDDot=off  SenseDistDDot=off  SenseIncDDot=off
  ArmB : PMIOPort  Side=Left
  EndEff : PMIOPort  Port=2  Side=Right
  wires:
  PS-Simulink Converter8/1 -> Mux1/3
  PS-Simulink Converter7/1 -> Mux1/2
  PS-Simulink Converter6/1 -> Mux1/1
  Mux1/1 -> Terminator/1  "endEffPos"
  connections:
  Transform Sensor/RConn1 -- EndEff/RConn1
  PS-Simulink Converter8/LConn1 -- Transform Sensor/RConn4
  PS-Simulink Converter7/LConn1 -- Transform Sensor/RConn3
  PS-Simulink Converter6/LConn1 -- Transform Sensor/RConn2
  ArmB/RConn1 -- Transform Sensor/LConn1

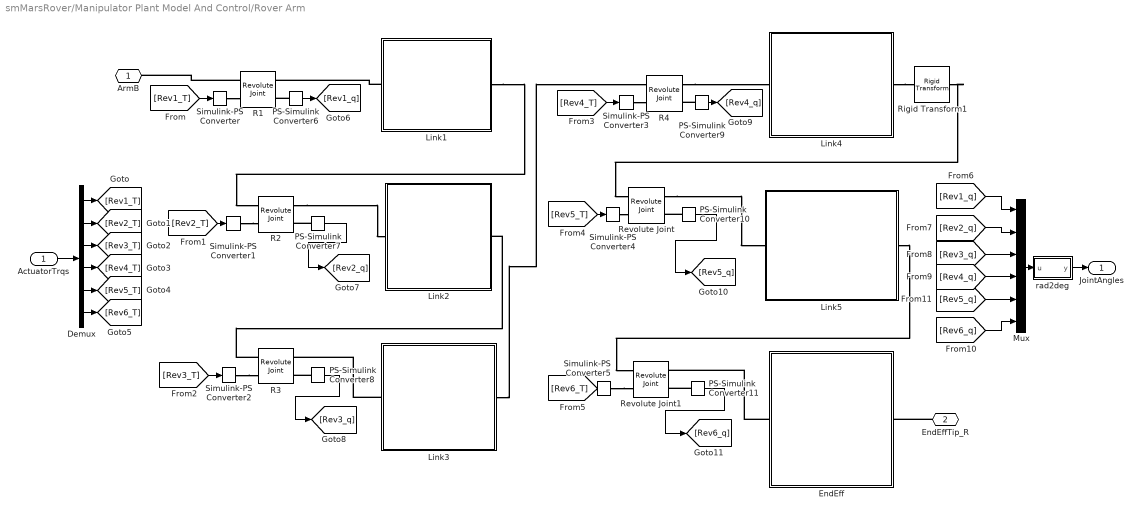
== system smMarsRover/Manipulator Plant Model And Control/Rover Arm ==
  ActuatorTrqs : Inport
  Demux : Demux  Outputs=6
  EndEff : Subsystem
      mask Display: image('$imagefile'); % Use "Edit Image" on toolstrip to change.
  Link1 : Subsystem
      mask Display: image('$imagefile'); % Use "Edit Image" on toolstrip to change.
  Link2 : Subsystem
      mask Display: image('$imagefile'); % Use "Edit Image" on toolstrip to change.
  Link3 : Subsystem
      mask Display: image('$imagefile'); % Use "Edit Image" on toolstrip to change.
  Link4 : Subsystem
      mask Display: image('$imagefile'); % Use "Edit Image" on toolstrip to change.
  Link5 : Subsystem
      mask Display: image('$imagefile'); % Use "Edit Image" on toolstrip to change.
  Mux : Mux  Inputs=6
  PS-Simulink Converter{6..11} (6 alike) : nesl_utility/PS-Simulink Converter  PhysicalDomain=network_engine_domain  SubClassName=ps_output  LeftPortType=input  RightPortType=output  PseudoPeriodic=off  Frequencies=[]  VectorFormat=1-D array  Unit=inherit  AffineConversion=off
  R1 : sm_lib/Joints/Revolute Joint  JointMode=Normal  CompositeWrenchDir=FollowerOnBase  CompositeWrenchFrame=BaseFrame  SenseConstraintForce=off  SenseConstraintTorque=off  SenseTotalForce=off  SenseTotalTorque=off  PositionTargetSpecify=on  PositionTargetPriority=High  PositionTargetValue=arm_q0(1)  PositionTargetValueUnits=deg  VelocityTargetSpecify=off  VelocityTargetPriority=High  VelocityTargetValue=0  VelocityTargetValueUnits=deg/s  EquilibriumPosition=0  EquilibriumPositionUnits=deg  SpringStiffness=0  SpringStiffnessUnits=N*m/deg  DampingCoefficient=D  DampingCoefficientUnits=N*m/(deg/s)  LowerLimitSpecify=off  LowerLimitBound=-90  LowerLimitBoundUnits=deg  LowerLimitStiffness=1e4  LowerLimitStiffnessUnits=N*m/deg  LowerLimitDamping=10  LowerLimitDampingUnits=N*m/(deg/s)  LowerLimitTransitionRegionWidth=0.1  LowerLimitTransitionRegionWidthUnits=deg  UpperLimitSpecify=off  UpperLimitBound=90  UpperLimitBoundUnits=deg  UpperLimitStiffness=1e4  UpperLimitStiffnessUnits=N*m/deg  UpperLimitDamping=10  UpperLimitDampingUnits=N*m/(deg/s)  UpperLimitTransitionRegionWidth=0.1  UpperLimitTransitionRegionWidthUnits=deg  TorqueActuationMode=InputTorque  MotionActuationMode=ComputedMotion  SensePosition=on  SenseVelocity=off  SenseAcceleration=off  SenseTorqueForce=off  SenseLowerLimitTorqueForce=off  SenseUpperLimitTorqueForce=off
  R2 : sm_lib/Joints/Revolute Joint  JointMode=Normal  CompositeWrenchDir=FollowerOnBase  CompositeWrenchFrame=BaseFrame  SenseConstraintForce=off  SenseConstraintTorque=off  SenseTotalForce=off  SenseTotalTorque=off  PositionTargetSpecify=on  PositionTargetPriority=High  PositionTargetValue=arm_q0(2)  PositionTargetValueUnits=deg  VelocityTargetSpecify=off  VelocityTargetPriority=High  VelocityTargetValue=0  VelocityTargetValueUnits=deg/s  EquilibriumPosition=0  EquilibriumPositionUnits=deg  SpringStiffness=0  SpringStiffnessUnits=N*m/deg  DampingCoefficient=D  DampingCoefficientUnits=N*m/(deg/s)  LowerLimitSpecify=off  LowerLimitBound=-90  LowerLimitBoundUnits=deg  LowerLimitStiffness=1e4  LowerLimitStiffnessUnits=N*m/deg  LowerLimitDamping=10  LowerLimitDampingUnits=N*m/(deg/s)  LowerLimitTransitionRegionWidth=0.1  LowerLimitTransitionRegionWidthUnits=deg  UpperLimitSpecify=off  UpperLimitBound=90  UpperLimitBoundUnits=deg  UpperLimitStiffness=1e4  UpperLimitStiffnessUnits=N*m/deg  UpperLimitDamping=10  UpperLimitDampingUnits=N*m/(deg/s)  UpperLimitTransitionRegionWidth=0.1  UpperLimitTransitionRegionWidthUnits=deg  TorqueActuationMode=InputTorque  MotionActuationMode=ComputedMotion  SensePosition=on  SenseVelocity=off  SenseAcceleration=off  SenseTorqueForce=off  SenseLowerLimitTorqueForce=off  SenseUpperLimitTorqueForce=off
  R3 : sm_lib/Joints/Revolute Joint  JointMode=Normal  CompositeWrenchDir=FollowerOnBase  CompositeWrenchFrame=BaseFrame  SenseConstraintForce=off  SenseConstraintTorque=off  SenseTotalForce=off  SenseTotalTorque=off  PositionTargetSpecify=on  PositionTargetPriority=High  PositionTargetValue=arm_q0(3)  PositionTargetValueUnits=deg  VelocityTargetSpecify=off  VelocityTargetPriority=High  VelocityTargetValue=0  VelocityTargetValueUnits=deg/s  EquilibriumPosition=0  EquilibriumPositionUnits=deg  SpringStiffness=0  SpringStiffnessUnits=N*m/deg  DampingCoefficient=D  DampingCoefficientUnits=N*m/(deg/s)  LowerLimitSpecify=off  LowerLimitBound=-10  LowerLimitBoundUnits=deg  LowerLimitStiffness=1e4  LowerLimitStiffnessUnits=N*m/deg  LowerLimitDamping=10  LowerLimitDampingUnits=N*m/(deg/s)  LowerLimitTransitionRegionWidth=0.1  LowerLimitTransitionRegionWidthUnits=deg  UpperLimitSpecify=off  UpperLimitBound=160  UpperLimitBoundUnits=deg  UpperLimitStiffness=1e4  UpperLimitStiffnessUnits=N*m/deg  UpperLimitDamping=10  UpperLimitDampingUnits=N*m/(deg/s)  UpperLimitTransitionRegionWidth=0.1  UpperLimitTransitionRegionWidthUnits=deg  TorqueActuationMode=InputTorque  MotionActuationMode=ComputedMotion  SensePosition=on  SenseVelocity=off  SenseAcceleration=off  SenseTorqueForce=off  SenseLowerLimitTorqueForce=off  SenseUpperLimitTorqueForce=off
  R4 : sm_lib/Joints/Revolute Joint  JointMode=Normal  CompositeWrenchDir=FollowerOnBase  CompositeWrenchFrame=BaseFrame  SenseConstraintForce=off  SenseConstraintTorque=off  SenseTotalForce=off  SenseTotalTorque=off  PositionTargetSpecify=on  PositionTargetPriority=High  PositionTargetValue=arm_q0(4)  PositionTargetValueUnits=deg  VelocityTargetSpecify=off  VelocityTargetPriority=High  VelocityTargetValue=0  VelocityTargetValueUnits=deg/s  EquilibriumPosition=0  EquilibriumPositionUnits=deg  SpringStiffness=0  SpringStiffnessUnits=N*m/deg  DampingCoefficient=D  DampingCoefficientUnits=N*m/(deg/s)  LowerLimitSpecify=off  LowerLimitBound=-90  LowerLimitBoundUnits=deg  LowerLimitStiffness=1e4  LowerLimitStiffnessUnits=N*m/deg  LowerLimitDamping=10  LowerLimitDampingUnits=N*m/(deg/s)  LowerLimitTransitionRegionWidth=0.1  LowerLimitTransitionRegionWidthUnits=deg  UpperLimitSpecify=off  UpperLimitBound=90  UpperLimitBoundUnits=deg  UpperLimitStiffness=1e4  UpperLimitStiffnessUnits=N*m/deg  UpperLimitDamping=10  UpperLimitDampingUnits=N*m/(deg/s)  UpperLimitTransitionRegionWidth=0.1  UpperLimitTransitionRegionWidthUnits=deg  TorqueActuationMode=InputTorque  MotionActuationMode=ComputedMotion  SensePosition=on  SenseVelocity=off  SenseAcceleration=off  SenseTorqueForce=off  SenseLowerLimitTorqueForce=off  SenseUpperLimitTorqueForce=off
  Revolute Joint : sm_lib/Joints/Revolute Joint  JointMode=Normal  CompositeWrenchDir=FollowerOnBase  CompositeWrenchFrame=BaseFrame  SenseConstraintForce=off  SenseConstraintTorque=off  SenseTotalForce=off  SenseTotalTorque=off  PositionTargetSpecify=on  PositionTargetPriority=High  PositionTargetValue=arm_q0(5)  PositionTargetValueUnits=deg  VelocityTargetSpecify=off  VelocityTargetPriority=High  VelocityTargetValue=0  VelocityTargetValueUnits=deg/s  EquilibriumPosition=0  EquilibriumPositionUnits=deg  SpringStiffness=0  SpringStiffnessUnits=N*m/deg  DampingCoefficient=D2  DampingCoefficientUnits=N*m/(deg/s)  LowerLimitSpecify=off  LowerLimitBound=-90  LowerLimitBoundUnits=deg  LowerLimitStiffness=1e4  LowerLimitStiffnessUnits=N*m/deg  LowerLimitDamping=10  LowerLimitDampingUnits=N*m/(deg/s)  LowerLimitTransitionRegionWidth=0.1  LowerLimitTransitionRegionWidthUnits=deg  UpperLimitSpecify=off  UpperLimitBound=90  UpperLimitBoundUnits=deg  UpperLimitStiffness=1e4  UpperLimitStiffnessUnits=N*m/deg  UpperLimitDamping=10  UpperLimitDampingUnits=N*m/(deg/s)  UpperLimitTransitionRegionWidth=0.1  UpperLimitTransitionRegionWidthUnits=deg  TorqueActuationMode=InputTorque  MotionActuationMode=ComputedMotion  SensePosition=on  SenseVelocity=off  SenseAcceleration=off  SenseTorqueForce=off  SenseLowerLimitTorqueForce=off  SenseUpperLimitTorqueForce=off
  Revolute Joint1 : sm_lib/Joints/Revolute Joint  JointMode=Normal  CompositeWrenchDir=FollowerOnBase  CompositeWrenchFrame=BaseFrame  SenseConstraintForce=off  SenseConstraintTorque=off  SenseTotalForce=off  SenseTotalTorque=off  PositionTargetSpecify=on  PositionTargetPriority=High  PositionTargetValue=arm_q0(6)  PositionTargetValueUnits=deg  VelocityTargetSpecify=off  VelocityTargetPriority=High  VelocityTargetValue=0  VelocityTargetValueUnits=deg/s  EquilibriumPosition=0  EquilibriumPositionUnits=deg  SpringStiffness=0  SpringStiffnessUnits=N*m/deg  DampingCoefficient=D2  DampingCoefficientUnits=N*m/(deg/s)  LowerLimitSpecify=off  LowerLimitBound=-90  LowerLimitBoundUnits=deg  LowerLimitStiffness=1e4  LowerLimitStiffnessUnits=N*m/deg  LowerLimitDamping=10  LowerLimitDampingUnits=N*m/(deg/s)  LowerLimitTransitionRegionWidth=0.1  LowerLimitTransitionRegionWidthUnits=deg  UpperLimitSpecify=off  UpperLimitBound=90  UpperLimitBoundUnits=deg  UpperLimitStiffness=1e4  UpperLimitStiffnessUnits=N*m/deg  UpperLimitDamping=10  UpperLimitDampingUnits=N*m/(deg/s)  UpperLimitTransitionRegionWidth=0.1  UpperLimitTransitionRegionWidthUnits=deg  TorqueActuationMode=InputTorque  MotionActuationMode=ComputedMotion  SensePosition=on  SenseVelocity=off  SenseAcceleration=off  SenseTorqueForce=off  SenseLowerLimitTorqueForce=off  SenseUpperLimitTorqueForce=off
  Rigid Transform1 : sm_lib/Frames and Transforms/Rigid Transform  RotationMethod=None  FollAlignAxisA=+X  BaseAlignAxisA=+Y  FollAlignAxisB=+Y  BaseAlignAxisB=+Z  RotationStandardAxis=+X  RotationAngle=90  RotationAngleUnits=deg  RotationArbitraryAxis=[0 0 1]  RotationSequenceAxes=FollowerAxes  RotationSequence=XYX  RotationSequenceAngles=[0 0 0]  RotationSequenceAnglesUnits=deg  RotationMatrix=[1 0 0; 0 1 0; 0 0 1]  Quaternion=[1 0 0 0]  TranslationMethod=StandardAxis  TranslationCartesianOffset=[0 0 0]  TranslationCartesianOffsetUnits=cm  TranslationStandardAxis=+Z  TranslationStandardOffset=3  TranslationStandardOffsetUnits=cm  TranslationROffset=0  TranslationROffsetUnits=m  TranslationThetaOffset=0  TranslationThetaOffsetUnits=deg  TranslationZOffset=0  TranslationZOffsetUnits=m
  Simulink-PS Converter{,1..5} (6 alike) : nesl_utility/Simulink-PS Converter  PhysicalDomain=network_engine_domain  SubClassName=ps_input  LeftPortType=input  RightPortType=output  PseudoPeriodic=off  Frequencies=[]  NoiseDistribution=none  NoiseParameters=[]  Unit=1  AffineConversion=off  FilteringAndDerivatives=provide  SimscapeFilterOrder=1  InputFilterTimeConstant=0.001  UdotUserProvided=0
  rad2deg : MATLAB Function  TreatAsAtomicUnit=on
  ArmB : PMIOPort  Side=Left
  EndEffTip_R : PMIOPort  Port=2  Side=Left
  JointAngles : Outport
  wires:
  Mux/1 -> rad2deg/1(u)
  [Rev2_q] -> Mux/2
  [Rev3_q] -> Mux/3
  [Rev4_q] -> Mux/4
  [Rev5_q] -> Mux/5
  [Rev6_q] -> Mux/6
  ActuatorTrqs/1 -> Demux/1
  Demux/1 -> [Rev1_T]
  Demux/2 -> [Rev2_T]
  Demux/3 -> [Rev3_T]
  Demux/4 -> [Rev4_T]
  Demux/5 -> [Rev5_T]
  Demux/6 -> [Rev6_T]
  [Rev1_T] -> Simulink-PS Converter/1
  [Rev2_T] -> Simulink-PS Converter1/1
  [Rev3_T] -> Simulink-PS Converter2/1
  [Rev4_T] -> Simulink-PS Converter3/1
  [Rev5_T] -> Simulink-PS Converter4/1
  [Rev6_T] -> Simulink-PS Converter5/1
  PS-Simulink Converter6/1 -> [Rev1_q]
  PS-Simulink Converter7/1 -> [Rev2_q]
  PS-Simulink Converter8/1 -> [Rev3_q]
  PS-Simulink Converter9/1 -> [Rev4_q]
  PS-Simulink Converter10/1 -> [Rev5_q]
  PS-Simulink Converter11/1 -> [Rev6_q]
  rad2deg/1(y) -> JointAngles/1
  [Rev1_q] -> Mux/1
  connections:
  Link1/LConn1 -- R1/RConn1
  Link3/RConn1 -- R4/LConn1
  R2/RConn1 -- Link2/LConn1
  R3/LConn1 -- Link2/RConn1
  R4/RConn1 -- Link4/LConn1
  Link1/RConn1 -- R2/LConn1
  Link3/LConn1 -- R3/RConn1
  Link4/RConn1 -- Rigid Transform1/LConn1
  EndEff/LConn1 -- Revolute Joint1/RConn1
  Rigid Transform1/RConn1 -- Revolute Joint/LConn1
  EndEffTip_R/RConn1 -- EndEff/RConn1
  R1/LConn1 -- ArmB/RConn1
  Link5/RConn1 -- Revolute Joint1/LConn1
  Revolute Joint/RConn1 -- Link5/LConn1
  Simulink-PS Converter/RConn1 -- R1/LConn2
  Simulink-PS Converter1/RConn1 -- R2/LConn2
  Simulink-PS Converter2/RConn1 -- R3/LConn2
  Simulink-PS Converter3/RConn1 -- R4/LConn2
  Simulink-PS Converter4/RConn1 -- Revolute Joint/LConn2
  Simulink-PS Converter5/RConn1 -- Revolute Joint1/LConn2
  PS-Simulink Converter6/LConn1 -- R1/RConn2
  PS-Simulink Converter7/LConn1 -- R2/RConn2
  PS-Simulink Converter8/LConn1 -- R3/RConn2
  PS-Simulink Converter9/LConn1 -- R4/RConn2
  PS-Simulink Converter10/LConn1 -- Revolute Joint/RConn2
  PS-Simulink Converter11/LConn1 -- Revolute Joint1/RConn2
